simulink model "ex2_1"  (Simulink 7.5)
settings: Solver=ode45  StartTime=0.0  StopTime=10.0  RelTol=1e-3
libraries: powerlib x10, powerlib_extras x7
settings Model: Creator=107108103  LastModifiedBy=Sambhav
settings OptimizationCC: InitFltsAndDblsToZero=on
settings DebuggingCC: StrictBusMsg=Warning

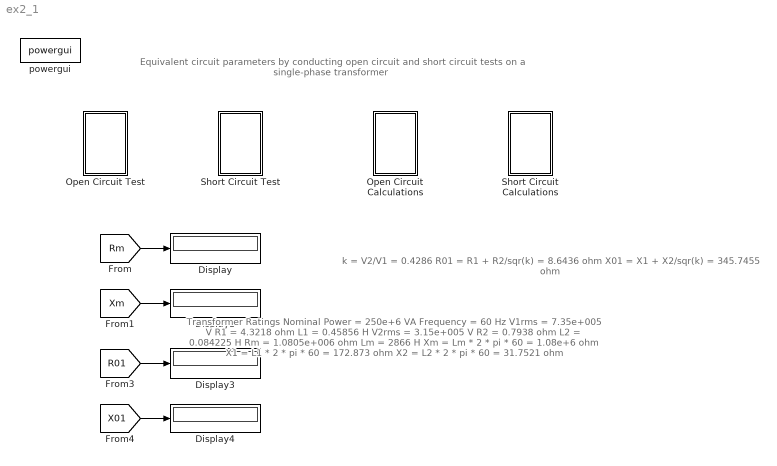
== system ex2_1 ==
  note: Transformer Ratings
      | Nominal Power = 250e+6 VA
      | Frequency = 60 Hz
      | V1rms = 7.35e+005 V
      | R1 = 4.3218 ohm
      | L1 = 0.45856 H
      | V2rms = 3.15e+005 V
      | R2 = 0.7938 ohm
      | L2 = 0.084225 H
      | Rm = 1.0805e+006 ohm
      | Lm = 2866 H
      | Xm = Lm * 2 * pi * 60 = 1.08e+6 ohm
      | X1 = L1 * 2 * pi * 60 = 172.873 ohm
      | X2 = L2 * 2 * pi * 60 = 31.7521 ohm
  note: k = V2/V1 = 0.4286
      | R01 = R1 + R2/sqr(k)
      | = 8.6436 ohm
      | X01 = X1 + X2/sqr(k)
      | = 345.7455 ohm
  note: Equivalent circuit parameters by conducting open circuit and
      | short circuit tests on a single-phase transformer
  Display{,1,3..4} (4 alike) : Display
  Open Circuit Calculations : Subsystem
  Open Circuit Test : Subsystem
  Short Circuit Calculations : Subsystem
  Short Circuit Test : Subsystem
  powergui : powerlib/powergui  SystemSampleTime=-1  SimulationMode=Continuous  SampleTime=50e-6  frequency=60  SPID=off  DisableSnubberDevices=off  DisableRonSwitches=off  DisableVfSwitches=off  SwTol=0  Interpol=off  frequencyindice=60  echomessages=off  HookPort=off  DisplayEquations=off  FunctionMessages=off  EnableUseOfTLC=off  x0status=blocks  RestoreLinks=warning  ResistiveCurrentMeasurement=off  Frange=[0:2:500]  Ylog=off  Xlog=on  ShowGrid=off  save=off  variable=ZData  ZoomFFT=on  StartTime=0.0  cycles=1  DisplayStyle=1  fundamental=60  FreqAxis=off  MaxFrequency=1000  frequencyindicesteady=1  RmsSteady=1  display=off  Ts=0  methode=off
  wires:
  [Rm] -> Display/1
  [Xm] -> Display1/1
  [R01] -> Display3/1
  [X01] -> Display4/1

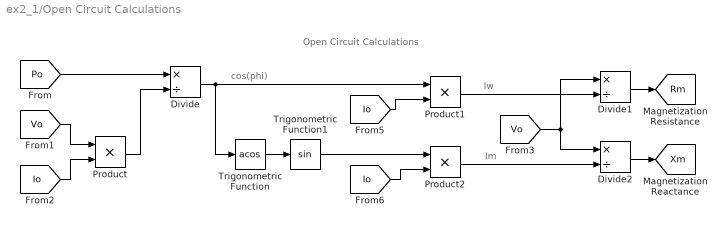
== system ex2_1/Open Circuit Calculations ==
  note: Iw
  note: Im
  note: cos(phi)
  note: Open Circuit Calculations
  Divide : Product  Inputs=*/  OutDataType=sfix(16)  OutScaling=2^-10
  Divide1 : Product  Inputs=*/  OutDataType=sfix(16)  OutScaling=2^-10
  Divide2 : Product  Inputs=*/  OutDataType=sfix(16)  OutScaling=2^-10
  Product : Product  OutDataType=sfix(16)  OutScaling=2^0  RndMeth=Zero
  Product1 : Product  OutDataType=sfix(16)  OutScaling=2^0  RndMeth=Zero
  Product2 : Product  OutDataType=sfix(16)  OutScaling=2^0  RndMeth=Zero
  Trigonometric Function : Trigonometry  Operator=acos
  Trigonometric Function1 : Trigonometry
  tag scope: Rm=global, Xm=global
  wires:
  [Vo] -> Product/1
  [Io] -> Product/2
  [Po] -> Divide/1
  Product/1 -> Divide/2
  [Vo] -> Divide1/1, Divide2/1
  [Io] -> Product1/2
  [Io] -> Product2/2
  Divide/1 -> Trigonometric Function/1, Product1/1
  Product1/1 -> Divide1/2
  Product2/1 -> Divide2/2
  Trigonometric Function/1 -> Trigonometric Function1/1
  Trigonometric Function1/1 -> Product2/1
  Divide2/1 -> [Xm]
  Divide1/1 -> [Rm]

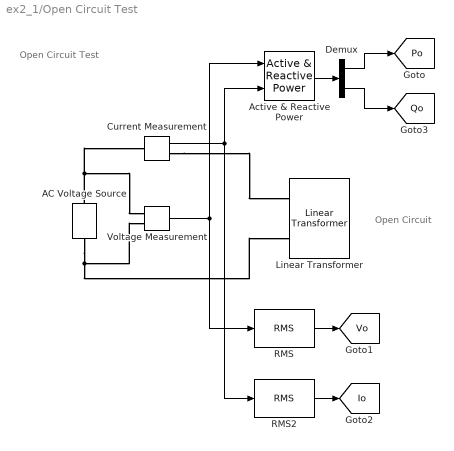
== system ex2_1/Open Circuit Test ==
  note: Open Circuit
  note: Open Circuit Test
  AC Voltage Source : powerlib/Electrical Sources/AC Voltage Source  DialogController=POWERSYS.PowerSysDialog  SystemSampleTime=-1  Amplitude=(3.15e+005)*sqrt(2)  Phase=0  Frequency=60  SampleTime=0  Measurements=None
  Active & Reactive Power : powerlib_extras/Measurements/Active & Reactive Power  DialogController=POWERSYS.PowerSysDialog  SystemSampleTime=-1  f1=60
  Current Measurement : powerlib/Measurements/Current Measurement  DialogController=POWERSYS.PowerSysDialog  SystemSampleTime=-1  PhasorSimulation=off  OutputType=Complex  PSBequivalent=0
  Demux : Demux  Outputs=2
  Linear Transformer : powerlib/Elements/Linear Transformer  DialogController=POWERSYS.PowerSysDialog  PhysicalDomain=powersysdomain  SubClassName=unknown  LeftPortType=p1  RightPortType=p1  LConnTagsString=a|b  RConnTagsString=A|B  UNITS=SI  NominalPower=[ 250e6 60 ]  winding1=[7.35e+005 4.3218 0.45856]  winding2=[3.15e+005 0.7938 0.084225]  ThreeWindings=off  winding3=[3.15e+005 0.7938 0.084225]  RmLm=[1.0805e+006 2866]  Measurements=None  DataType=on
  RMS : powerlib_extras/Measurements/RMS  DialogController=POWERSYS.PowerSysDialog  SystemSampleTime=-1  f1=60
  RMS2 : powerlib_extras/Measurements/RMS  DialogController=POWERSYS.PowerSysDialog  SystemSampleTime=-1  f1=60
  Voltage Measurement : powerlib/Measurements/Voltage Measurement  DialogController=POWERSYS.PowerSysDialog  SystemSampleTime=-1  PhasorSimulation=off  OutputType=Complex  PSBequivalent=0
  tag scope: Io=global, Po=global, Qo=global, Vo=global
  wires:
  RMS/1 -> [Vo]
  RMS2/1 -> [Io]
  Demux/1 -> [Po]
  Demux/2 -> [Qo]
  Active & Reactive Power/1 -> Demux/1
  Voltage Measurement/1 -> Active & Reactive Power/1, RMS/1
  Current Measurement/1 -> Active & Reactive Power/2, RMS2/1
  connections:
  AC Voltage Source/LConn1 -- Linear Transformer/LConn2 -- Voltage Measurement/LConn2
  AC Voltage Source/RConn1 -- Current Measurement/LConn1 -- Voltage Measurement/LConn1
  Current Measurement/RConn1 -- Linear Transformer/LConn1

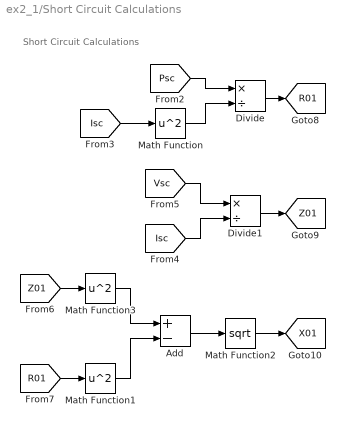
== system ex2_1/Short Circuit Calculations ==
  note: Short Circuit Calculations
  Add : Sum  Inputs=+-  OutDataType=sfix(16)  OutScaling=2^-10
  Divide : Product  Inputs=*/  OutDataType=sfix(16)  OutScaling=2^-10
  Divide1 : Product  Inputs=*/  OutDataType=sfix(16)  OutScaling=2^-10
  Math Function : Math  Operator=square  OutDataType=sfix(16)  OutScaling=2^0  SaturateOnIntegerOverflow=on
  Math Function1 : Math  Operator=square  OutDataType=sfix(16)  OutScaling=2^0  SaturateOnIntegerOverflow=on
  Math Function2 : Math  Operator=sqrt  OutDataType=sfix(16)  OutScaling=2^0  SaturateOnIntegerOverflow=on
  Math Function3 : Math  Operator=square  OutDataType=sfix(16)  OutScaling=2^0  SaturateOnIntegerOverflow=on
  tag scope: R01=global, X01=global, Z01=global
  wires:
  [Psc] -> Divide/1
  [Isc] -> Math Function/1
  Math Function/1 -> Divide/2
  Divide/1 -> [R01]
  [Vsc] -> Divide1/1
  [Isc] -> Divide1/2
  Divide1/1 -> [Z01]
  Math Function2/1 -> [X01]
  Add/1 -> Math Function2/1
  Math Function3/1 -> Add/1
  Math Function1/1 -> Add/2
  [Z01] -> Math Function3/1
  [R01] -> Math Function1/1

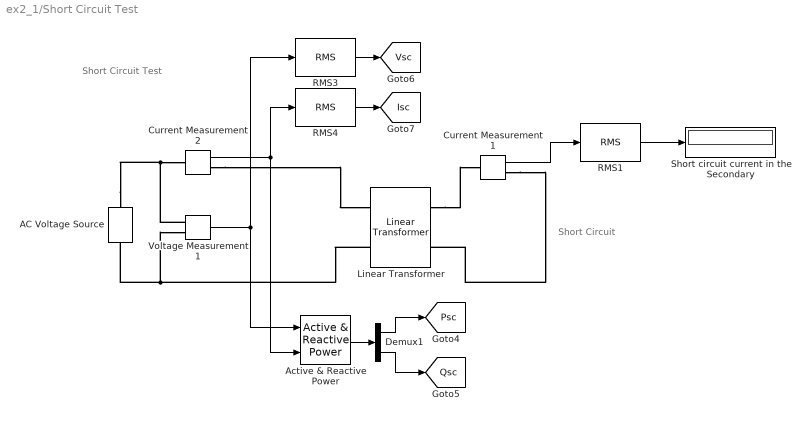
== system ex2_1/Short Circuit Test ==
  note: Short Circuit Test
  note: Short Circuit
  AC Voltage Source : powerlib/Electrical Sources/AC Voltage Source  DialogController=POWERSYS.PowerSysDialog  SystemSampleTime=-1  Amplitude=(1.2e+005)*sqrt(2)  Phase=0  Frequency=60  SampleTime=0  Measurements=None
  Active & Reactive Power : powerlib_extras/Measurements/Active & Reactive Power  DialogController=POWERSYS.PowerSysDialog  SystemSampleTime=-1  f1=60
  Current Measurement1 : powerlib/Measurements/Current Measurement  DialogController=POWERSYS.PowerSysDialog  SystemSampleTime=-1  PhasorSimulation=off  OutputType=Complex  PSBequivalent=0
  Current Measurement2 : powerlib/Measurements/Current Measurement  DialogController=POWERSYS.PowerSysDialog  SystemSampleTime=-1  PhasorSimulation=off  OutputType=Complex  PSBequivalent=0
  Demux1 : Demux  Outputs=2
  Linear Transformer : powerlib/Elements/Linear Transformer  DialogController=POWERSYS.PowerSysDialog  PhysicalDomain=powersysdomain  SubClassName=unknown  LeftPortType=p1  RightPortType=p1  LConnTagsString=a|b  RConnTagsString=A|B  UNITS=SI  NominalPower=[ 250e6 60 ]  winding1=[7.35e+005 4.3218 0.45856]  winding2=[3.15e+005 0.7938 0.084225]  ThreeWindings=off  winding3=[3.15e+005 0.7938 0.084225]  RmLm=[1.0805e+006 2866]  Measurements=None  DataType=on
  RMS1 : powerlib_extras/Measurements/RMS  DialogController=POWERSYS.PowerSysDialog  SystemSampleTime=-1  f1=60
  RMS3 : powerlib_extras/Measurements/RMS  DialogController=POWERSYS.PowerSysDialog  SystemSampleTime=-1  f1=60
  RMS4 : powerlib_extras/Measurements/RMS  DialogController=POWERSYS.PowerSysDialog  SystemSampleTime=-1  f1=60
  Short circuit current in the Secondary : Display
  Voltage Measurement1 : powerlib/Measurements/Voltage Measurement  DialogController=POWERSYS.PowerSysDialog  SystemSampleTime=-1  PhasorSimulation=off  OutputType=Complex  PSBequivalent=0
  tag scope: Isc=global, Psc=global, Qsc=global, Vsc=global
  wires:
  RMS1/1 -> Short circuit current in the Secondary/1
  Current Measurement1/1 -> RMS1/1
  Active & Reactive Power/1 -> Demux1/1
  Voltage Measurement1/1 -> Active & Reactive Power/1, RMS3/1
  Current Measurement2/1 -> Active & Reactive Power/2, RMS4/1
  Demux1/1 -> [Psc]
  Demux1/2 -> [Qsc]
  RMS3/1 -> [Vsc]
  RMS4/1 -> [Isc]
  connections:
  AC Voltage Source/LConn1 -- Linear Transformer/LConn2 -- Voltage Measurement1/LConn2
  AC Voltage Source/RConn1 -- Voltage Measurement1/LConn1 -- Current Measurement2/LConn1
  Linear Transformer/RConn1 -- Current Measurement1/LConn1
  Current Measurement1/RConn1 -- Linear Transformer/RConn2
  Current Measurement2/RConn1 -- Linear Transformer/LConn1
